simulink model "mizan_plant"  (R2024b)
settings: Solver=ode1  StartTime=0.0  StopTime=86400  FixedStep=60  RelTol=1e-3
libraries: fl_lib x5, nesl_utility x3
settings Model: Creator=Nouman  LastModifiedBy=Nouman

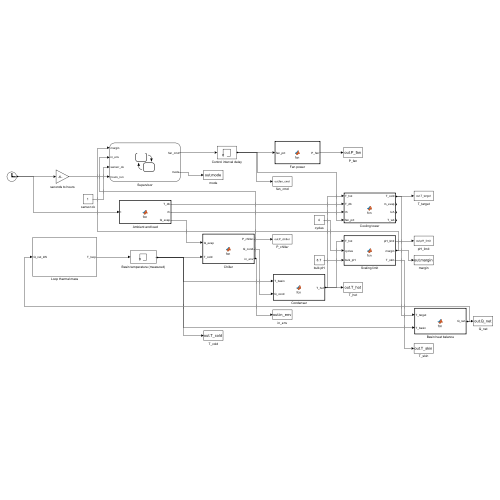
[thumbnail: Simulink's stored preview of the top-level diagram]
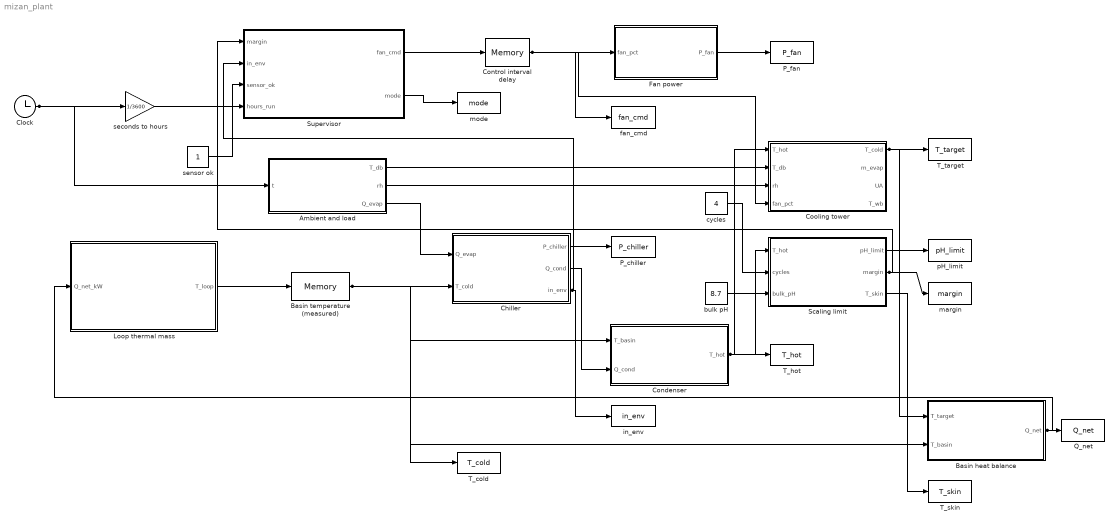
== system mizan_plant ==
  Ambient and load : MATLAB Function  TreatAsAtomicUnit=on
  Basin heat balance : MATLAB Function  TreatAsAtomicUnit=on
  Basin temperature (measured) : Memory  InitialCondition=26.85
  Chiller : MATLAB Function  TreatAsAtomicUnit=on
  Clock : Clock
  Condenser : MATLAB Function  TreatAsAtomicUnit=on
  Control interval delay : Memory  InitialCondition=85
  Cooling tower : MATLAB Function  TreatAsAtomicUnit=on
  Fan power : MATLAB Function  TreatAsAtomicUnit=on
  Loop thermal mass : Subsystem
  P_chiller : ToWorkspace  VariableName=P_chiller  SaveFormat=Timeseries  SampleTime=-1
  P_fan : ToWorkspace  VariableName=P_fan  SaveFormat=Timeseries  SampleTime=-1
  Q_net : ToWorkspace  VariableName=Q_net  SaveFormat=Timeseries  SampleTime=-1
  Scaling limit : MATLAB Function  TreatAsAtomicUnit=on
  Supervisor : Stateflow chart  TreatAsAtomicUnit=on
  T_cold : ToWorkspace  VariableName=T_cold  SaveFormat=Timeseries  SampleTime=-1
  T_hot : ToWorkspace  VariableName=T_hot  SaveFormat=Timeseries  SampleTime=-1
  T_skin : ToWorkspace  VariableName=T_skin  SaveFormat=Timeseries  SampleTime=-1
  T_target : ToWorkspace  VariableName=T_target  SaveFormat=Timeseries  SampleTime=-1
  bulk pH : Constant  Value=8.7
  cycles : Constant  Value=4
  fan_cmd : ToWorkspace  VariableName=fan_cmd  SaveFormat=Timeseries  SampleTime=-1
  in_env : ToWorkspace  VariableName=in_env  SaveFormat=Timeseries  SampleTime=-1
  margin : ToWorkspace  VariableName=margin  SaveFormat=Timeseries  SampleTime=-1
  mode : ToWorkspace  VariableName=mode  SaveFormat=Timeseries  SampleTime=-1
  pH_limit : ToWorkspace  VariableName=pH_limit  SaveFormat=Timeseries  SampleTime=-1
  seconds to hours : Gain  Gain=1/3600
  sensor ok : Constant
  wires:
  Clock/1 -> Ambient and load/1(t), seconds to hours/1
  seconds to hours/1 -> Supervisor/4(hours_run)
  bulk pH/1 -> Scaling limit/3(bulk_pH)
  Supervisor/2(mode) -> mode/1
  Supervisor/1(fan_cmd) -> Control interval delay/1
  sensor ok/1 -> Supervisor/3(sensor_ok)
  Basin heat balance/1(Q_net) -> Loop thermal mass/1(Q_net_kW), Q_net/1
  Loop thermal mass/1(T_loop) -> Basin temperature (measured)/1
  Ambient and load/2(rh) -> Cooling tower/3(rh)
  Ambient and load/3(Q_evap) -> Chiller/1(Q_evap)
  Ambient and load/1(T_db) -> Cooling tower/2(T_db)
  Basin temperature (measured)/1 -> Condenser/1(T_basin), Basin heat balance/2(T_basin), Chiller/2(T_cold), T_cold/1
  Control interval delay/1 -> Cooling tower/4(fan_pct), Fan power/1(fan_pct), fan_cmd/1
  Scaling limit/2(margin) -> Supervisor/1(margin), margin/1
  Chiller/2(Q_cond) -> Condenser/2(Q_cond)
  Chiller/1(P_chiller) -> P_chiller/1
  Chiller/3(in_env) -> Supervisor/2(in_env), in_env/1
  Fan power/1(P_fan) -> P_fan/1
  cycles/1 -> Scaling limit/2(cycles)
  Condenser/1(T_hot) -> Cooling tower/1(T_hot), Scaling limit/1(T_hot), T_hot/1
  Cooling tower/1(T_cold) -> Basin heat balance/1(T_target), T_target/1
  Scaling limit/1(pH_limit) -> pH_limit/1
  Scaling limit/3(T_skin) -> T_skin/1

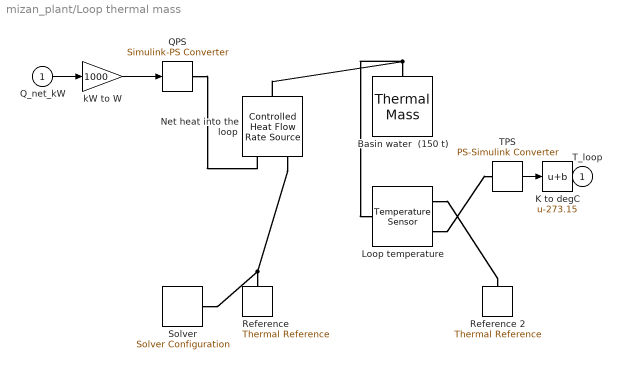
== system mizan_plant/Loop thermal mass ==
  Q_net_kW : Inport
  Basin water  (150 t) : fl_lib/Thermal/Thermal Elements/Thermal Mass  mass_type=foundation.enum.constant_variable.constant  mass=1.5e5 kg  sp_heat=4186 J/(K*kg)  mass_min=1e-6 kg  num_ports=foundation.enum.numPorts2.one  m_specify=off  m_priority=High  m=1 kg  m_nominal_specify=off  m_nominal_value=1  m_nominal_unit=kg  T_specify=off  T_priority=High  T=300 K  T_nominal_specify=off  T_nominal_value=1  T_nominal_unit=K  Q_specify=off  Q_priority=None  Q=0 W  Q_nominal_specify=off  Q_nominal_value=1  Q_nominal_unit=W
  K to degC : Bias  Bias=-273.15  SaturateOnIntegerOverflow=off
  Loop temperature : fl_lib/Thermal/Thermal Sensors/Temperature Sensor  temperature_measure=foundation.enum.MeasurementReference.difference
  Net heat into the loop : fl_lib/Thermal/Thermal Sources/Controlled Heat Flow Rate Source
  QPS : nesl_utility/Simulink-PS Converter  PhysicalDomain=network_engine_domain  SubClassName=ps_input  LeftPortType=input  RightPortType=output  PseudoPeriodic=off  Frequencies=[]  NoiseDistribution=none  NoiseParameters=[]  Unit=1  AffineConversion=off  FilteringAndDerivatives=provide  SimscapeFilterOrder=1  InputFilterTimeConstant=0.001  UdotUserProvided=0
  Reference : fl_lib/Thermal/Thermal Elements/Thermal Reference
  Reference 2 : fl_lib/Thermal/Thermal Elements/Thermal Reference
  Solver : nesl_utility/Solver Configuration  PhysicalDomain=network_engine_domain  SubClassName=solver  LeftPortType=input  RightPortType=generic  Tones=[]  Harmonics=[]  SimulateNoise=off  Profile=off  UseLocalSampling=off  EnableSwitchedLinearOptims=on  FrequencyDomain=off  UseCCode=off  RelTol=0.001  AbsTol=0.001  MinStep=1e-09  ToWorkspace=off  RevertToSquareIcSolve=off  NumHomotopyIterations=100  PhasorMode=off  PhasorModeNumHarmonics=1  ConsistencySolver=NEWTON_XTOL_AFTER_FTOL  IndexReductionMethod=DerivativeReplacement  DoDC=off  ResidualTolerance=1e-09  ConsistencyTolSource=GLOBAL  ConsistencyAbsTol=0.001  ConsistencyRelTol=0.001  ConsistencyTolFactor=0.001  UseLocalSolver=on  LocalSolverChoice=NE_BACKWARD_EULER_ADVANCER  ResolveIndetEquations=on  FunctionEvalNumThread=1  LocalSolverSampleTime=60  DoFixedCost=off  MaxNonlinIter=3  MaxModeIter=2  ComputeImpulses=off  ImpulseIterations=2  LinearAlgebra=auto  LinearAlgebraNumThread=0  EquationFormulation=NE_TIME_EF  DelaysMemoryBudget=1024  AutomaticFiltering=on  FilteringTimeConstant=0.001  PartitionStorageMethod=AS_NEEDED  PartitionMemoryBudget=1024  PartitionMethod=ROBUST  MultibodyUseLocalSolver=off  MultibodyLocalSolverChoice=ODE1  MultibodyLocalSolverSampleTime=0.001
  TPS : nesl_utility/PS-Simulink Converter  PhysicalDomain=network_engine_domain  SubClassName=ps_output  LeftPortType=input  RightPortType=output  PseudoPeriodic=off  Frequencies=[]  VectorFormat=inherit  Unit=inherit  AffineConversion=off
  kW to W : Gain  Gain=1000
  T_loop : Outport
  wires:
  Q_net_kW/1 -> kW to W/1
  kW to W/1 -> QPS/1
  TPS/1 -> K to degC/1
  K to degC/1 -> T_loop/1
  connections:
  QPS/RConn1 -- Net heat into the loop/RConn1
  Basin water  (150 t)/LConn1 -- Net heat into the loop/LConn1 -- Loop temperature/LConn1
  Reference/LConn1 -- Net heat into the loop/RConn2 -- Solver/RConn1
  Loop temperature/RConn1 -- Reference 2/LConn1
  Loop temperature/RConn2 -- TPS/LConn1

== matlab function mizan_plant/Cooling tower ==
  data: T_hot input; T_cold output; T_db input; rh input; fan_pct input; m_evap output; UA output; T_wb output
function [T_cold, m_evap, UA, T_wb] = fcn(T_hot, T_db, rh, fan_pct)
% The tower, from the validated Poppe heat-and-mass-transfer model.
% Returns the cold water it can reach, the evaporation rate, an
% equivalent conductance UA [kW/K] for the physical network, and the
% wet-bulb -- the coldest temperature the tower could ever reach.
coder.extrinsic('mizan_tower_step');
T_cold = 30; m_evap = 0; UA = 100; T_wb = 25;
[T_cold, m_evap, UA, T_wb] = mizan_tower_step(T_hot, T_db, rh, fan_pct);

== matlab function mizan_plant/Ambient and load ==
  data: t input; T_db output; rh output; Q_evap output
function [T_db, rh, Q_evap] = fcn(t)
% One Dhahran summer day: cool before dawn, brutal in the afternoon, with
% the cooling load following the heat as it does in every real plant.
hr = mod(t/3600, 24);
s  = sin(pi*max(hr-6,0)/16)^2;
T_db   = 32 + 12*s;              % 32 C at night, 44 C at peak
rh     = 0.55 - 0.25*s;          % drier as it heats
Q_evap = 10000*(0.62 + 0.38*s);  % kW of cooling delivered

== matlab function mizan_plant/Chiller ==
  data: Q_evap input; P_chiller output; T_cold input; Q_cond output; in_env output
function [P_chiller, Q_cond, in_env] = fcn(Q_evap, T_cold)
% Electrical power drawn by the chiller, and the heat the tower must
% therefore reject: the cooling load PLUS the compressor work.
%
% IN_ENV is 0 when entering condenser water leaves the range the
% manufacturer's curves were fitted in. Left unchecked an optimiser walks
% out of that range and collects a saving that does not exist. This one
% did exactly that once, and booked a false water saving on the strength
% of it.
coder.extrinsic('mizan_chiller_step');
P_chiller = 1500; in_env = 1;
[P_chiller, in_env] = mizan_chiller_step(Q_evap, T_cold);
Q_cond = Q_evap + P_chiller;

== matlab function mizan_plant/Scaling limit ==
  data: T_hot input; pH_limit output; cycles input; bulk_pH input; margin output; T_skin output
function [pH_limit, margin, T_skin] = fcn(T_hot, cycles, bulk_pH)
% The pH above which magnesium silicate deposits, evaluated at the
% CONDENSER TUBE SKIN rather than in the bulk water.
%
% Brucite's saturation pH is RETROGRADE -- it falls as the surface gets
% hotter -- so the same loop is safe at low load and depositing at high
% load, with pH and conductivity reading identical in both cases. No
% fixed setpoint can express that.
coder.extrinsic('mizan_chem_step');
pH_limit = 9; T_skin = 40;
[pH_limit, T_skin] = mizan_chem_step(T_hot, cycles);
% An extrinsic call is opaque to the compiler, so the result is forced
% real and finite here. The chemistry can legitimately return an infinite
% limit when there is no magnesium in the water, and a solver transient
% can briefly ask for a temperature no water reaches.
pH_limit = real(pH_limit);
if ~isfinite(pH_limit), pH_limit = 14; end
T_skin   = real(T_skin);
margin = pH_limit - bulk_pH;   % positive = safe, negative = depositing

== matlab function mizan_plant/Condenser ==
  data: T_basin input; T_hot output; Q_cond input
function T_hot = fcn(T_basin, Q_cond)
% Water leaves the tower basin cold, picks up the condenser duty, and
% arrives back at the top of the tower hot:
%
%     T_hot = T_basin + Q_cond / (m_w * cp)
%
% That temperature rise is the condenser RANGE, and it is what sets the
% tube skin temperature -- which is where the scale actually forms.
m_w = 478;  cp = 4.186;
T_hot = T_basin + Q_cond/(m_w*cp);

== matlab function mizan_plant/Basin heat balance ==
  data: T_target input; Q_net output; T_basin input
function Q_net = fcn(T_target, T_basin)
% The tower basin is a mixing volume. Water arrives in it at whatever
% temperature the tower managed to reach, at the circulating flow rate,
% and the basin's own temperature relaxes towards that:
%
%     M cp dT/dt = m_w cp (T_target - T_basin)
%
% The time constant is the basin inventory over the circulating flow --
% about five minutes here -- and it is the reason a condenser loop cannot
% be controlled as though it responded instantly.
m_w = 478;  cp = 4.186;
Q_net = m_w*cp*(T_target - T_basin);

== stateflow chart mizan_plant/Supervisor ==
  state SHADOW
    du:
    mode = 1;
    fan_cmd = 85;
  state ADVISORY
    du:
    mode = 2;
    fan_cmd = 85;
  state FALLBACK
    du:
    mode = 0;
    fan_cmd = 85;
  state CLOSED_LOOP
    du:
    mode = 3;
    fan_cmd = 85 - 25*tanh(max(-margin,0)*8);
  (default) -> SHADOW
  FALLBACK -> ADVISORY : [sensor_ok && in_env]
  SHADOW -> ADVISORY : [hours_run > 1344]
  ADVISORY -> FALLBACK [order 2] : [~sensor_ok]
  CLOSED_LOOP -> FALLBACK : [~sensor_ok || ~in_env]
  ADVISORY -> CLOSED_LOOP [order 1] : [hours_run > 1512]
  data: margin input; in_env input; sensor_ok input; hours_run input; fan_cmd output; mode output

== matlab function mizan_plant/Fan power ==
  data: fan_pct input; P_fan output
function P_fan = fcn(fan_pct)
% Fan shaft power by the affinity law -- power goes as the CUBE of air
% flow, which is why backing the fan off is the single biggest lever the
% controller has on tower energy.
P_fan = 110*(max(min(fan_pct,100),0)/100)^3;
